simulink model "ident_pend_EV3"  (R2019b)
settings: Solver=ode1  StartTime=0.0  StopTime=30  FixedStep=h  RelTol=1e-3  EnableMultiTasking=on
libraries: legoev3lib x4
settings Model: SimulationMode=external  ExtModeTrigDuration=2  Creator=kawata  LastModifiedBy=Noritaka Okayasu
settings DataIOCC: LimitDataPoints=on  SaveFormat=Array  ReturnWorkspaceOutputs=off
settings OptimizationCC: LifeSpan=1  EfficientTunableParamExpr=on
settings DebuggingCC: UnderspecifiedInitializationDetection=Classic  MergeDetectMultiDrivingBlocksExec=none  SFUnexpectedBacktrackingDiag=warning  SFNoUnconditionalDefaultTransitionDiag=warning  SFExecutionAtInitializationDiag=none  ArithmeticOperatorsInVariantConditions=warning
settings HardwareCC: ProdBitPerPointer=32  ProdBitPerSizeT=32  ProdBitPerPtrDiffT=32  ProdLargestAtomicInteger=Long  ProdIntDivRoundTo=Undefined  ProdWordSize=32  ProdHWDeviceType=ARM Compatible->ARM 9
settings ModelReferenceCC: PropagateSignalLabelsOutOfModel=off
settings SFSimCC: SimUseLocalCustomCode=off  MATLABDynamicMemAlloc=off  CustomCodeUndefinedFunction=UseInterfaceOnly
settings RTWCC: Description=Run on Target Hardware  SystemTargetFile=realtime.tlc  GenerateMakefile=off  TemplateMakefile=realtime.tmf  RTWVerbose=off  RTWUseLocalCustomCode=off
settings CodeAppCC: StateflowObjectComments=on
settings STFCustomTargetCC: TargetLibSuffix=.a  GenerateSampleERTMain=on  ERTCustomFileBanners=on  SupportNonInlinedSFcns=off  RemoveResetFunc=on  SupportVariableSizeSignals=on  MATLABClassNameForMDSCustomization=Simulink.SoftwareTarget.ERTCustomization  SystemTargetFile=realtime.tlc
settings ERTTargetCC: MultiwordLength=2048  GenerateSampleERTMain=on  ParMdlRefBuildCompliant=off  CompOptLevelCompliant=off  ConcurrentExecutionCompliant=off  CombineOutputUpdateFcns=off  SupportContinuousTime=on  SupportVariableSizeSignals=on  ModelStepFunctionPrototypeControlCompliant=off  CPPClassGenCompliant=off  UseToolchainInfoCompliant=off  ExtMode=on  ExtModeMexArgs='192.168.11.5' 0 17725 5  ERTSrcFileBannerTemplate=realtime_code_template.cgt  ERTHdrFileBannerTemplate=realtime_code_template.cgt  ERTDataSrcFileTemplate=realtime_code_template.cgt  ERTDataHdrFileTemplate=realtime_code_template.cgt  ERTCustomFileTemplate=realtime_file_process.tlc  ConvertIfToSwitch=off  SuppressUnreachableDefaultCases=off
settings ConfigComp: CovMetricSettings=dw  CovHtmlReporting=on  CovSaveCumulativeToWorkspaceVar=on  CovSaveSingleToWorkspaceVar=on  CovExternalEMLEnable=off  CovSFcnEnable=off

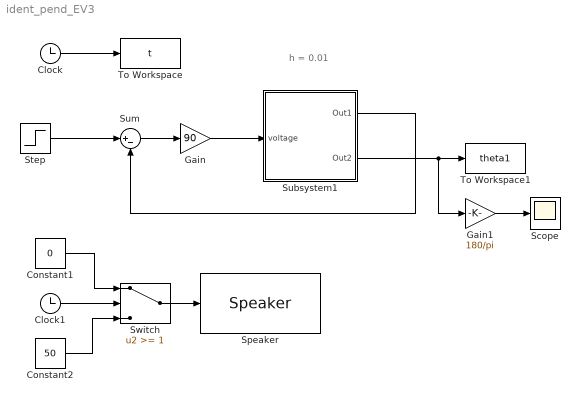
== system ident_pend_EV3 ==
  note: h = 0.01
  Clock : Clock
  Clock1 : Clock
  Constant1 : Constant  Value=0
  Constant2 : Constant  Value=50
  Gain : Gain  Gain=90
  Gain1 : Gain  Gain=180/pi
  Scope : Scope
  Speaker : legoev3lib/Speaker  sinputMode=Volume only  sspeakerFreq=100  sspeakerVolume=50  sspeakerDuration=1000
      settings: SourceProductName=Simulink Support Package for LEGO MINDSTORMS EV3 Hardware  SourceProductBaseCode=LEGOEV3
  Step : Step  After=pi/3  SampleTime=0
  Subsystem1 : Subsystem
  Sum : Sum  Inputs=|+-
  Switch : Switch  Threshold=1
  To Workspace : ToWorkspace  VariableName=t  SampleTime=-1
  To Workspace1 : ToWorkspace  VariableName=theta1  SampleTime=-1
  wires:
  Clock/1 -> To Workspace/1
  Clock1/1 -> Switch/2
  Switch/1 -> Speaker/1
  Constant1/1 -> Switch/1
  Constant2/1 -> Switch/3
  Gain/1 -> Subsystem1/1(voltage)
  Sum/1 -> Gain/1
  Subsystem1/1(Out1) -> Sum/2
  Subsystem1/2(Out2) -> Gain1/1, To Workspace1/1
  Gain1/1 -> Scope/1
  Step/1 -> Sum/1

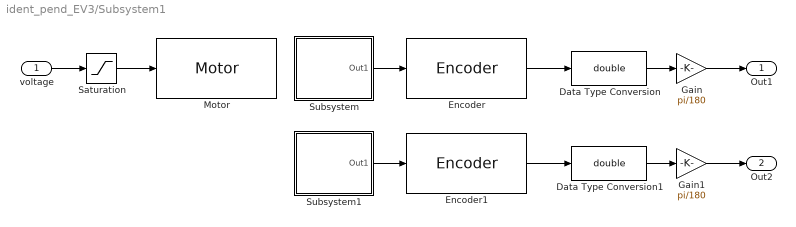
== system ident_pend_EV3/Subsystem1 ==
  voltage : Inport
  Data Type Conversion : DataTypeConversion  OutDataTypeStr=double
  Data Type Conversion1 : DataTypeConversion  OutDataTypeStr=double
  Encoder : legoev3lib/Encoder  portNumber=A  opMode=Reset by external signal  sampleTime=h
      settings: SourceProductName=Simulink Support Package for LEGO MINDSTORMS EV3 Hardware  SourceProductBaseCode=LEGOEV3
  Encoder1 : legoev3lib/Encoder  portNumber=C  opMode=Reset by external signal  sampleTime=h
      settings: SourceProductName=Simulink Support Package for LEGO MINDSTORMS EV3 Hardware  SourceProductBaseCode=LEGOEV3
  Gain : Gain  Gain=pi/180
  Gain1 : Gain  Gain=pi/180
  Motor : legoev3lib/Motor  sportNumber=A  sstopAction=Brake
  Saturation : Saturate  UpperLimit=100  LowerLimit=-100
  Subsystem : Subsystem
  Subsystem1 : Subsystem
  Out1 : Outport
  Out2 : Outport  Port=2
  wires:
  Gain1/1 -> Out2/1
  Subsystem1/1(Out1) -> Encoder1/1
  Data Type Conversion1/1 -> Gain1/1
  Encoder1/1 -> Data Type Conversion1/1
  Saturation/1 -> Motor/1
  Gain/1 -> Out1/1
  Subsystem/1(Out1) -> Encoder/1
  Data Type Conversion/1 -> Gain/1
  Encoder/1 -> Data Type Conversion/1
  voltage/1 -> Saturation/1

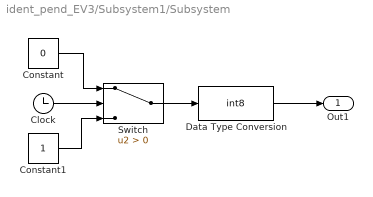
== system ident_pend_EV3/Subsystem1/Subsystem ==
  Clock : Clock
  Constant : Constant  Value=0
  Constant1 : Constant
  Data Type Conversion : DataTypeConversion  OutDataTypeStr=int8  RndMeth=Simplest
  Switch : Switch  Criteria=u2 > Threshold
  Out1 : Outport
  wires:
  Data Type Conversion/1 -> Out1/1
  Constant1/1 -> Switch/3
  Constant/1 -> Switch/1
  Switch/1 -> Data Type Conversion/1
  Clock/1 -> Switch/2

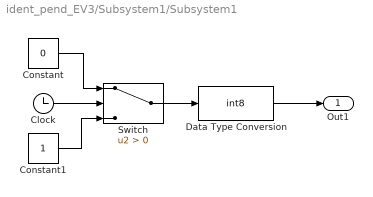
== system ident_pend_EV3/Subsystem1/Subsystem1 ==
  Clock : Clock
  Constant : Constant  Value=0
  Constant1 : Constant
  Data Type Conversion : DataTypeConversion  OutDataTypeStr=int8  RndMeth=Simplest
  Switch : Switch  Criteria=u2 > Threshold
  Out1 : Outport
  wires:
  Clock/1 -> Switch/2
  Switch/1 -> Data Type Conversion/1
  Constant/1 -> Switch/1
  Constant1/1 -> Switch/3
  Data Type Conversion/1 -> Out1/1
